simulink model "Accelerator_Pedal_Position_Sensor"  (R2024a)
settings: Solver=VariableStepAuto  StartTime=0.0  StopTime=10.0  RelTol=1e-3
settings Model: Creator=DELL  LastModifiedBy=DELL
settings DataIOCC: LoadExternalInput=on

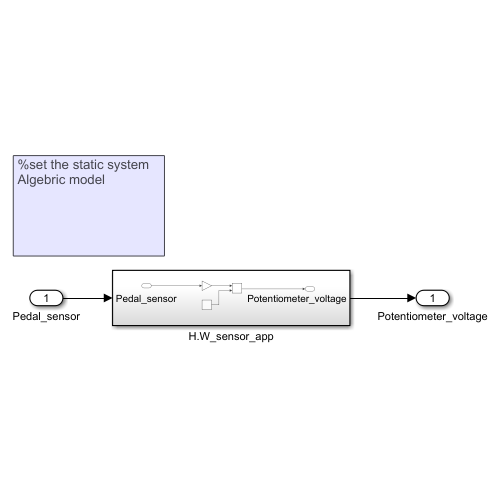
[thumbnail: Simulink's stored preview of the top-level diagram]
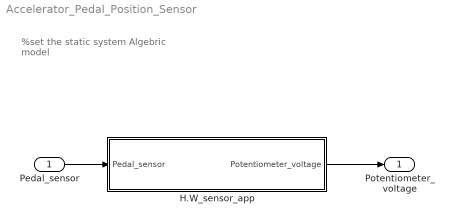
== system Accelerator_Pedal_Position_Sensor ==
  note: %set the static system
      | Algebric model
  Pedal_sensor : Inport
  H.W_sensor_app : Subsystem
  Potentiometer_voltage : Outport
  wires:
  Pedal_sensor/1 -> H.W_sensor_app/1(Pedal_sensor)
  H.W_sensor_app/1(Potentiometer_voltage) -> Potentiometer_voltage/1

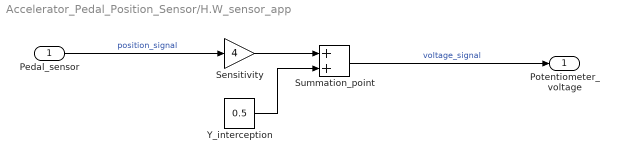
== system Accelerator_Pedal_Position_Sensor/H.W_sensor_app ==
  Pedal_sensor : Inport
  Sensitivity : Gain  Gain=4
  Summation_point : Sum
  Y_interception : Constant  Value=0.5
  Potentiometer_voltage : Outport
  wires:
  Y_interception/1 -> Summation_point/2
  Pedal_sensor/1 -> Sensitivity/1  "position_signal"
  Summation_point/1 -> Potentiometer_voltage/1  "voltage_signal"
  Sensitivity/1 -> Summation_point/1
